simulink library "TOWER_MASTER"  (Simulink 8.8)
settings: Solver=ode45  StartTime=0.0  StopTime=10.0  RelTol=1e-3  EnableMultiTasking=on
undefined symbols (not defined in the file): AC, AC2THRESHOLD, BF_WD_MASTER, GAS_WD_MASTER, GASAC, SIXOSEM_F_WD_AC_MASTER
libraries: cdsEpicsOut x163, cdsFilt x111, cdsTP x68, cdsFiltCtrl x56, cdsEpicsIn x47, cdsMuxMatrix x14, cdsRms x14, TOWER_MASTER x11, STATE_BIO_MASTER x8, cdsEpicsBinIn x6, cdsFunctionCall x4, VIS_LIB x2
(part 2 of 19)

== system TOWER_MASTER/common_blocks/BIOENCODE ==
  note: 1st - 16th bit
  note: 17th bit
  BIO_CTRL_In : Inport
  DIO_OUT : cdsEpicsOut/Subsystem  Tag=cdsEpicsOutput  Description=|
      | Purpose:                                          
      | Output a FE signal to an EPICS channel.           
      |                                                   
      | Operation:                                        
      | Takes input value and passes it to EPICS record.  
      |                                                   
      | Usage:                                            
      | Name the part with the desired EPICS rrecord name.
      settings: AttributesFormatString=%<Tag>
  Gain1 : Gain  Gain=65536
  Ground1 : Ground
  Sum : Sum
  WD_RESET : cdsEpicsBinIn/Subsystem  Tag=cdsEpicsBinIn  Description=|
      | Purpose:                                                                            
      | Create an EPICS binary (0 or 1) input channel to the FE realtime controls.          
      |                                                                                     
      | Operation:                                                                          
      | Outputs value from an EPICS ai record. Value is binary input (bi Epics record type).
      |                                                                                     
      | Usage:                                                                              
      | Name the part with the desired EPICS channel name.
      settings: AttributesFormatString=%<Tag>
  BIO_CTRL_Out : Outport
  wires:
  DIO_OUT/1 -> BIO_CTRL_Out/1
  Sum/1 -> DIO_OUT/1
  BIO_CTRL_In/1 -> Sum/1
  WD_RESET/1 -> Gain1/1
  Ground1/1 -> WD_RESET/1
  Gain1/1 -> Sum/2

== system TOWER_MASTER/common_blocks/GASMASTER ==
  note: #DAQ Channels
      | LVDTINF_GAS_IN1 2048
      | DAMP_GAS_IN1 2048
      | DAMP_GAS_OUT 256
  LVDT_GAS_In : Inport
  MODAL_In : Inport  Port=2
  PEM_SEIS_Z_In : Inport  Port=3
  COILOUT_CTRL : Inport  Port=4
  COILOUTF_MASK : Inport  Port=5
  MASTERSW_In : Inport  Port=6
  WDRESET_In : Inport  Port=7
  BLOCKFLAG : Inport  Port=8
  Modal_IN : Inport  Port=9
  ADD : Subsystem
  COILOUTF : Subsystem
  DAMP : Subsystem
  Demux9 : Demux
  LVDTINF : Subsystem
  MASTER : Subsystem
  Mux9 : Mux  Inputs=2
  SEISFF : Subsystem
  SENSCORR : Subsystem
  SET : Subsystem
  SUMOUT : Subsystem
  Sum1 : Sum  Inputs=++|
  Sum2 : Sum  Inputs=++|
  Sum5 : Sum  Inputs=-+|
  TEST : Subsystem
  Terminator2 : Terminator
  WATCHDOG : cdsFunctionCall/Subsystem  Tag=cdsFunctionCall  Description=inline OSEMWATCHDOG /opt/rtcds/userapps/release/vis/common/src/WATCHDOG.c
      settings: AttributesFormatString=%<Tag>\n%<Description>
  WD : Subsystem
  WDMON : TOWER_MASTER/common_blocks/WDMONMASTER
  GAS_CTR_Out : Outport
  GAS_INF_Out : Outport  Port=2
  WD_STAT_Out : Outport  Port=3
  DAMP_STAT_Out : Outport  Port=4
  wires:
  [FFSTATE] -> Terminator2/1
  SEISFF/1(SEIS_Out) -> ADD/1(SEISFF_In)
  SEISFF/2(SEIS_STATE_Out) -> [FFSTATE]
  PEM_SEIS_Z_In/1 -> SEISFF/1(SEIS_In), SENSCORR/1(SEIS_GAS_In)
  Sum1/1 -> Sum5/2, GAS_INF_Out/1
  SENSCORR/1(SC_GAS_Out) -> Sum1/1
  SET/1(GAS_Out) -> Sum5/1
  Sum5/1 -> DAMP/1(GAS_In)
  MODAL_In/1 -> ADD/2(MODAL_In)
  Demux9/2 -> WDMON/2
  Demux9/3 -> WDMON/3
  WD/1(GAS_AC_FLAG_Out) -> Mux9/2
  COILOUTF/1(Out1) -> MASTER/1(GAS_In)
  LVDTINF/1(Out1) -> Sum1/2
  WATCHDOG/1 -> Demux9/1
  Demux9/4 -> WDMON/4
  Mux9/1 -> WATCHDOG/1
  DAMP/2(DAMP_STATE_Out) -> [DAMPSTATE]
  DAMP/1(GAS_Out) -> ADD/4(DAMP_In)
  MASTERSW_In/1 -> MASTER/2(MASTERSWITCH)
  [WDBLOCKFLAG] -> WD_STAT_Out/1
  [DAMPSTATE] -> DAMP_STAT_Out/1
  TEST/1(GAS_Out) -> ADD/3(TEST_In)
  BLOCKFLAG/1 -> MASTER/3(BLOCKFLAG)
  MASTER/1(GAS_Out) -> GAS_CTR_Out/1
  ADD/1(GAS_MAIN_Out) -> SUMOUT/1(GAS_In)
  Demux9/1 -> WDMON/1, [WDBLOCKFLAG]
  LVDT_GAS_In/1 -> LVDTINF/1(In1), WD/1(GAS_In)
  COILOUT_CTRL/1 -> COILOUTF/2(In2)
  COILOUTF_MASK/1 -> COILOUTF/3(In3)
  WDRESET_In/1 -> Mux9/1
  SUMOUT/1(GAS_Out) -> Sum2/2
  Sum2/1 -> COILOUTF/1(In1)
  Modal_IN/1 -> Sum2/1

== system TOWER_MASTER/common_blocks/OKUTOMIGASMODAL ==
  F0GAS_In : Inport
  F1GAS_In : Inport  Port=2
  F2GAS_In : Inport  Port=3
  F3GAS_In : Inport  Port=4
  BFGAS_In : Inport  Port=5
  ADD : Subsystem
  DAMP : Subsystem
  Demux1 : Demux  Outputs=5
  Demux2 : Demux  Outputs=5
  LVDT2MODAL : cdsMuxMatrix/Subsystem  Tag=cdsMuxMatrix  Description=Any size matrix. Inputs and outputs must be connected using Mux and Demux parts.
      settings: AttributesFormatString=%<Tag>
  MODAL2COIL : cdsMuxMatrix/Subsystem  Tag=cdsMuxMatrix  Description=Any size matrix. Inputs and outputs must be connected using Mux and Demux parts.
      settings: AttributesFormatString=%<Tag>
  MODALOUT : Subsystem
  Mux1 : Mux  Inputs=5
  Mux2 : Mux  Inputs=5
  TEST : Subsystem
  Terminator1 : Terminator
  F0GAS_Out : Outport
  F1GAS_Out : Outport  Port=2
  F2GAS_Out : Outport  Port=3
  F3GAS_Out : Outport  Port=4
  BFGAS_Out : Outport  Port=5
  wires:
  MODALOUT/5(BF_Out) -> BFGAS_Out/1
  MODALOUT/4(F3_Out) -> F3GAS_Out/1
  MODALOUT/3(F2_Out) -> F2GAS_Out/1
  MODALOUT/1(F0_Out) -> F0GAS_Out/1
  MODALOUT/2(F1_Out) -> F1GAS_Out/1
  Demux1/5 -> MODALOUT/5(BF_In)
  Demux1/4 -> MODALOUT/4(F3_In)
  Demux1/3 -> MODALOUT/3(M2_In)
  Demux1/2 -> MODALOUT/2(F1_In)
  Demux1/1 -> MODALOUT/1(F0_In)
  Mux2/1 -> MODAL2COIL/1
  MODAL2COIL/1 -> Demux1/1
  ADD/5(M5_MAIN_Out) -> Mux2/5
  ADD/4(M4_MAIN_Out) -> Mux2/4
  ADD/1(M1_MAIN_Out) -> Mux2/1
  ADD/2(M2_MAIN_Out) -> Mux2/2
  ADD/3(M3_MAIN_Out) -> Mux2/3
  DAMP/1(M1_Out) -> ADD/6(DAMP_M1_In)
  DAMP/5(M5_Out) -> ADD/10(DAMP_M5_In)
  DAMP/2(M2_Out) -> ADD/7(DAMP_M2_In)
  DAMP/4(M4_Out) -> ADD/9(DAMP_M4_In)
  DAMP/3(M3_Out) -> ADD/8(DAMP_M3_In)
  DAMP/6(DAMP_STATE_Out) -> Terminator1/1
  Demux2/2 -> DAMP/2(M2_In)
  Demux2/3 -> DAMP/3(M3_In)
  Demux2/4 -> DAMP/4(M4_In)
  Demux2/1 -> DAMP/1(M1_In)
  Demux2/5 -> DAMP/5(M5_In)
  LVDT2MODAL/1 -> Demux2/1
  TEST/5(M5_Out) -> ADD/5(TEST_M5_In)
  TEST/4(M4_Out) -> ADD/4(TEST_M4_In)
  TEST/3(M3_Out) -> ADD/3(TEST_M3_In)
  TEST/2(M2_Out) -> ADD/2(TEST_M2_In)
  TEST/1(M1_Out) -> ADD/1(TEST_M1_In)
  F1GAS_In/1 -> Mux1/2
  F2GAS_In/1 -> Mux1/3
  BFGAS_In/1 -> Mux1/5
  F0GAS_In/1 -> Mux1/1
  F3GAS_In/1 -> Mux1/4
  Mux1/1 -> LVDT2MODAL/1

== system TOWER_MASTER/common_blocks/OKUTOMIKALMAN ==
  COIL_In1 : Inport
  COIL_In2 : Inport  Port=2
  MEAS_In1 : Inport  Port=3
  MEAS_In2 : Inport  Port=4
  A : cdsMuxMatrix/Subsystem  Tag=cdsMuxMatrix  Description=Any size matrix. Inputs and outputs must be connected using Mux and Demux parts.
      settings: AttributesFormatString=%<Tag>
  ADD_OUTPUT : Subsystem
  ADD_STATE : Subsystem
  B : cdsMuxMatrix/Subsystem  Tag=cdsMuxMatrix  Description=Any size matrix. Inputs and outputs must be connected using Mux and Demux parts.
      settings: AttributesFormatString=%<Tag>
  C : cdsMuxMatrix/Subsystem  Tag=cdsMuxMatrix  Description=Any size matrix. Inputs and outputs must be connected using Mux and Demux parts.
      settings: AttributesFormatString=%<Tag>
  D : cdsMuxMatrix/Subsystem  Tag=cdsMuxMatrix  Description=Any size matrix. Inputs and outputs must be connected using Mux and Demux parts.
      settings: AttributesFormatString=%<Tag>
  Demux{,1..3} (4 alike) : Demux  Outputs=6
  KEST : Subsystem
  Mux : Mux  Inputs=2
  Mux1 : Mux  Inputs=6
  Mux3 : Mux
  UnitDelay{,1..7} (8 alike) : UnitDelay
  Out1 : Outport
  Out2 : Outport  Port=2
  Out3 : Outport  Port=3
  Out4 : Outport  Port=4
  Out5 : Outport  Port=5
  Out6 : Outport  Port=6
  wires:
  KEST/3(X3_Out) -> Out3/1
  KEST/1(X1_Out) -> Out1/1
  KEST/6(X6_Out) -> Out6/1
  KEST/2(X2_Out) -> Out2/1
  KEST/4(X4_Out) -> Out4/1
  KEST/5(X5_Out) -> Out5/1
  ADD_OUTPUT/3(Xest_Out3) -> KEST/3(X3_In)
  ADD_OUTPUT/4(Xest_Out4) -> KEST/4(X4_In)
  ADD_OUTPUT/5(Xest_Out5) -> KEST/5(X5_In)
  ADD_OUTPUT/1(Xest_Out1) -> KEST/1(X1_In)
  ADD_OUTPUT/6(Xest_Out6) -> KEST/6(X6_In)
  ADD_OUTPUT/2(Xest_Out2) -> KEST/2(X2_In)
  MEAS_In2/1 -> Mux3/4
  MEAS_In1/1 -> Mux3/3
  Demux1/6 -> ADD_OUTPUT/12(C_In6)
  Demux1/1 -> ADD_OUTPUT/7(C_In1)
  Demux1/3 -> ADD_OUTPUT/9(C_In3)
  Demux1/2 -> ADD_OUTPUT/8(C_In2)
  Demux1/5 -> ADD_OUTPUT/11(C_In5)
  Demux1/4 -> ADD_OUTPUT/10(C_In4)
  Demux/6 -> ADD_OUTPUT/6(D_In6)
  Demux/3 -> ADD_OUTPUT/3(D_In3)
  Demux/2 -> ADD_OUTPUT/2(D_In2)
  Demux/4 -> ADD_OUTPUT/4(D_In4)
  Demux/5 -> ADD_OUTPUT/5(D_In5)
  Demux/1 -> ADD_OUTPUT/1(D_In1)
  Demux2/5 -> ADD_STATE/11(A_In5)
  Demux2/2 -> ADD_STATE/8(A_In2)
  Demux2/6 -> ADD_STATE/12(A_In6)
  Demux2/3 -> ADD_STATE/9(A_In3)
  Demux2/4 -> ADD_STATE/10(A_In4)
  Demux2/1 -> ADD_STATE/7(A_In1)
  Demux3/2 -> ADD_STATE/2(B_In2)
  Demux3/6 -> ADD_STATE/6(B_In6)
  Demux3/5 -> ADD_STATE/5(B_In5)
  Demux3/4 -> ADD_STATE/4(B_In4)
  Demux3/3 -> ADD_STATE/3(B_In3)
  Demux3/1 -> ADD_STATE/1(B_In1)
  COIL_In1/1 -> UnitDelay1/1, Mux3/1
  COIL_In2/1 -> UnitDelay2/1, Mux3/2
  ADD_STATE/6(dX_Out6) -> UnitDelay7/1
  ADD_STATE/5(dX_Out5) -> UnitDelay6/1
  ADD_STATE/4(dX_Out4) -> UnitDelay5/1
  ADD_STATE/3(dX_Out3) -> UnitDelay4/1
  ADD_STATE/2(dX_Out2) -> UnitDelay3/1
  ADD_STATE/1(dX_Out1) -> UnitDelay/1
  UnitDelay/1 -> Mux1/1
  UnitDelay7/1 -> Mux1/6
  UnitDelay6/1 -> Mux1/5
  UnitDelay3/1 -> Mux1/2
  UnitDelay4/1 -> Mux1/3
  UnitDelay5/1 -> Mux1/4
  UnitDelay1/1 -> Mux/1
  UnitDelay2/1 -> Mux/2
  B/1 -> Demux3/1
  Mux3/1 -> B/1
  A/1 -> Demux2/1
  Mux1/1 -> C/1, A/1
  Mux/1 -> D/1
  C/1 -> Demux1/1
  D/1 -> Demux/1

== system TOWER_MASTER/common_blocks/SHUTDOWNMASTER ==
  WD_Flag : Inport
  BLOCK : cdsEpicsOut/Subsystem  Tag=cdsEpicsOutput  Description=|
      | Purpose:                                          
      | Output a FE signal to an EPICS channel.           
      |                                                   
      | Operation:                                        
      | Takes input value and passes it to EPICS record.  
      |                                                   
      | Usage:                                            
      | Name the part with the desired EPICS rrecord name.
      settings: AttributesFormatString=%<Tag>
  CURRENTTRIG : cdsEpicsOut/Subsystem  Tag=cdsEpicsOutput  Description=|
      | Purpose:                                          
      | Output a FE signal to an EPICS channel.           
      |                                                   
      | Operation:                                        
      | Takes input value and passes it to EPICS record.  
      |                                                   
      | Usage:                                            
      | Name the part with the desired EPICS rrecord name.
      settings: AttributesFormatString=%<Tag>
  Demux : Demux
  FIRSTTRIG : cdsEpicsOut/Subsystem  Tag=cdsEpicsOutput  Description=|
      | Purpose:                                          
      | Output a FE signal to an EPICS channel.           
      |                                                   
      | Operation:                                        
      | Takes input value and passes it to EPICS record.  
      |                                                   
      | Usage:                                            
      | Name the part with the desired EPICS rrecord name.
      settings: AttributesFormatString=%<Tag>
  MODEL_RATE : cdsModelRate/Subsystem  Tag=cdsModelRate
      settings: AttributesFormatString=%<Tag>
  ModWD : cdsFunctionCall/Subsystem  Tag=cdsFunctionCall  Description=inline ModerateWD /opt/rtcds/userapps/release/vis/common/src/ModerateWD.c
      settings: AttributesFormatString=%<Tag>
  Mux : Mux  Inputs=3
  RAMPT : cdsEpicsIn/Subsystem  Tag=cdsEpicsIn  Description=|
      | Purpose:                                                                              
      | Create an EPICS input channel connection to the FE realtime controls.                 
      |                                                                                       
      | Operation:                                                                            
      | Outputs value from an EPICS ai record. Value is floating point with a precision of 3..
      |                                                                                       
      | Usage:                                                                                
      | Name the part with the desired EPICS channel name.
      settings: AttributesFormatString=%<Tag>
  STATE : cdsEpicsOut/Subsystem  Tag=cdsEpicsOutput  Description=|
      | Purpose:                                          
      | Output a FE signal to an EPICS channel.           
      |                                                   
      | Operation:                                        
      | Takes input value and passes it to EPICS record.  
      |                                                   
      | Usage:                                            
      | Name the part with the desired EPICS rrecord name.
      settings: AttributesFormatString=%<Tag>
  Terminator : Terminator
  Terminator1 : Terminator
  Block_Flag : Outport
  State : Outport  Port=2
  wires:
  Mux/1 -> ModWD/1
  ModWD/1 -> Demux/1
  MODEL_RATE/1 -> Mux/3
  BLOCK/1 -> Block_Flag/1
  WD_Flag/1 -> Mux/1
  CURRENTTRIG/1 -> Terminator1/1
  STATE/1 -> State/1
  Demux/3 -> FIRSTTRIG/1
  Demux/4 -> CURRENTTRIG/1
  Demux/2 -> STATE/1
  Demux/1 -> BLOCK/1
  FIRSTTRIG/1 -> Terminator/1
  RAMPT/1 -> Mux/2

== system TOWER_MASTER/common_blocks/WDMONMASTER ==
  BLOCK_Flag : Inport
  STATE_Flag : Inport  Port=2
  FIRST_Flag : Inport  Port=3
  CURRENT_Flag : Inport  Port=4
  BLOCK : cdsEpicsOut/Subsystem  Tag=cdsEpicsOutput  Description="field(PREC,\"3\")"
      settings: AttributesFormatString=%<Tag>
  CURRENTTRIG : cdsEpicsOut/Subsystem  Tag=cdsEpicsOutput  Description="field(PREC,\"3\")"
      settings: AttributesFormatString=%<Tag>
  FIRSTTRIG : cdsEpicsOut/Subsystem  Tag=cdsEpicsOutput  Description="field(PREC,\"3\")"
      settings: AttributesFormatString=%<Tag>
  STATE : cdsEpicsOut/Subsystem  Tag=cdsEpicsOutput  Description="field(PREC,\"3\")"
      settings: AttributesFormatString=%<Tag>
  Terminator{1,3,10..11} (4 alike) : Terminator
  wires:
  STATE_Flag/1 -> STATE/1
  FIRST_Flag/1 -> FIRSTTRIG/1
  CURRENT_Flag/1 -> CURRENTTRIG/1
  CURRENTTRIG/1 -> Terminator11/1
  FIRSTTRIG/1 -> Terminator10/1
  BLOCK_Flag/1 -> BLOCK/1
  BLOCK/1 -> Terminator1/1
  STATE/1 -> Terminator3/1

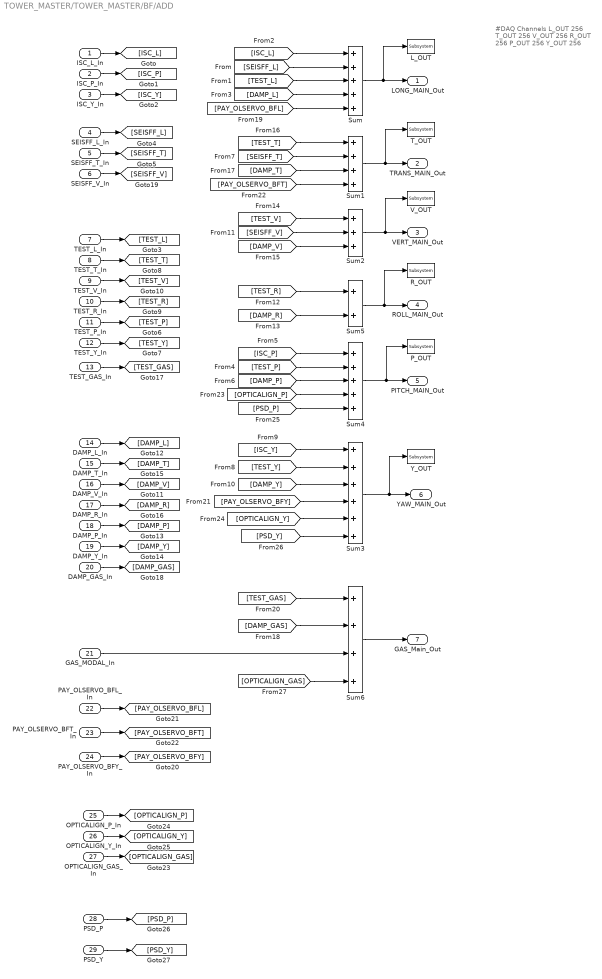
== system TOWER_MASTER/TOWER_MASTER/BF/ADD ==
  note: #DAQ Channels
      |
      | L_OUT 256
      | T_OUT 256
      | V_OUT 256
      | R_OUT 256
      | P_OUT 256
      | Y_OUT 256
  ISC_L_In : Inport
  ISC_P_In : Inport  Port=2
  ISC_Y_In : Inport  Port=3
  SEISFF_L_In : Inport  Port=4
  SEISFF_T_In : Inport  Port=5
  SEISFF_V_In : Inport  Port=6
  TEST_L_In : Inport  Port=7
  TEST_T_In : Inport  Port=8
  TEST_V_In : Inport  Port=9
  TEST_R_In : Inport  Port=10
  TEST_P_In : Inport  Port=11
  TEST_Y_In : Inport  Port=12
  TEST_GAS_In : Inport  Port=13
  DAMP_L_In : Inport  Port=14
  DAMP_T_In : Inport  Port=15
  DAMP_V_In : Inport  Port=16
  DAMP_R_In : Inport  Port=17
  DAMP_P_In : Inport  Port=18
  DAMP_Y_In : Inport  Port=19
  DAMP_GAS_In : Inport  Port=20
  GAS_MODAL_In : Inport  Port=21
  PAY_OLSERVO_BFL_In : Inport  Port=22
  PAY_OLSERVO_BFT_In : Inport  Port=23
  PAY_OLSERVO_BFY_In : Inport  Port=24
  OPTICALIGN_P_In : Inport  Port=25
  OPTICALIGN_Y_In : Inport  Port=26
  OPTICALIGN_GAS_In : Inport  Port=27
  PSD_P : Inport  Port=28
  PSD_Y : Inport  Port=29
  L_OUT : cdsTP/Subsystem  Tag=Test Point
      settings: AttributesFormatString=%<Tag>
  P_OUT : cdsTP/Subsystem  Tag=Test Point
      settings: AttributesFormatString=%<Tag>
  R_OUT : cdsTP/Subsystem  Tag=Test Point
      settings: AttributesFormatString=%<Tag>
  Sum : Sum  Inputs=+++++
  Sum1 : Sum  Inputs=++++
  Sum2 : Sum  Inputs=+++
  Sum3 : Sum  Inputs=++++++
  Sum4 : Sum  Inputs=+++++
  Sum5 : Sum
  Sum6 : Sum  Inputs=++++
  T_OUT : cdsTP/Subsystem  Tag=Test Point
      settings: AttributesFormatString=%<Tag>
  V_OUT : cdsTP/Subsystem  Tag=Test Point
      settings: AttributesFormatString=%<Tag>
  Y_OUT : cdsTP/Subsystem  Tag=Test Point
      settings: AttributesFormatString=%<Tag>
  LONG_MAIN_Out : Outport
  TRANS_MAIN_Out : Outport  Port=2
  VERT_MAIN_Out : Outport  Port=3
  ROLL_MAIN_Out : Outport  Port=4
  PITCH_MAIN_Out : Outport  Port=5
  YAW_MAIN_Out : Outport  Port=6
  GAS_Main_Out : Outport  Port=7
  wires:
  [PAY_OLSERVO_BFT] -> Sum1/4
  [PAY_OLSERVO_BFL] -> Sum/5
  PAY_OLSERVO_BFT_In/1 -> [PAY_OLSERVO_BFT]
  PAY_OLSERVO_BFL_In/1 -> [PAY_OLSERVO_BFL]
  GAS_MODAL_In/1 -> Sum6/3
  [DAMP_GAS] -> Sum6/2
  [TEST_GAS] -> Sum6/1
  [ISC_Y] -> Sum3/1
  [TEST_Y] -> Sum3/2
  [DAMP_Y] -> Sum3/3
  [PAY_OLSERVO_BFY] -> Sum3/4
  [DAMP_P] -> Sum4/3
  [TEST_P] -> Sum4/2
  [SEISFF_V] -> Sum2/2
  [SEISFF_T] -> Sum1/2
  [SEISFF_L] -> Sum/2
  Sum3/1 -> Y_OUT/1, YAW_MAIN_Out/1
  PAY_OLSERVO_BFY_In/1 -> [PAY_OLSERVO_BFY]
  [DAMP_V] -> Sum2/3
  [TEST_V] -> Sum2/1
  [DAMP_T] -> Sum1/3
  [TEST_T] -> Sum1/1
  [DAMP_R] -> Sum5/2
  [TEST_R] -> Sum5/1
  [ISC_P] -> Sum4/1
  ISC_Y_In/1 -> [ISC_Y]
  ISC_P_In/1 -> [ISC_P]
  ISC_L_In/1 -> [ISC_L]
  SEISFF_T_In/1 -> [SEISFF_T]
  SEISFF_L_In/1 -> [SEISFF_L]
  Sum1/1 -> T_OUT/1, TRANS_MAIN_Out/1
  Sum2/1 -> V_OUT/1, VERT_MAIN_Out/1
  Sum5/1 -> R_OUT/1, ROLL_MAIN_Out/1
  [DAMP_L] -> Sum/4
  [TEST_L] -> Sum/3
  [ISC_L] -> Sum/1
  Sum/1 -> L_OUT/1, LONG_MAIN_Out/1
  Sum4/1 -> P_OUT/1, PITCH_MAIN_Out/1
  Sum6/1 -> GAS_Main_Out/1
  SEISFF_V_In/1 -> [SEISFF_V]
  TEST_L_In/1 -> [TEST_L]
  TEST_T_In/1 -> [TEST_T]
  TEST_V_In/1 -> [TEST_V]
  TEST_R_In/1 -> [TEST_R]
  TEST_P_In/1 -> [TEST_P]
  TEST_Y_In/1 -> [TEST_Y]
  TEST_GAS_In/1 -> [TEST_GAS]
  DAMP_L_In/1 -> [DAMP_L]
  DAMP_T_In/1 -> [DAMP_T]
  DAMP_V_In/1 -> [DAMP_V]
  DAMP_R_In/1 -> [DAMP_R]
  DAMP_P_In/1 -> [DAMP_P]
  DAMP_Y_In/1 -> [DAMP_Y]
  DAMP_GAS_In/1 -> [DAMP_GAS]
  OPTICALIGN_Y_In/1 -> [OPTICALIGN_Y]
  OPTICALIGN_P_In/1 -> [OPTICALIGN_P]
  OPTICALIGN_GAS_In/1 -> [OPTICALIGN_GAS]
  PSD_P/1 -> [PSD_P]
  PSD_Y/1 -> [PSD_Y]
  [OPTICALIGN_P] -> Sum4/4
  [PSD_P] -> Sum4/5
  [OPTICALIGN_Y] -> Sum3/5
  [PSD_Y] -> Sum3/6
  [OPTICALIGN_GAS] -> Sum6/4

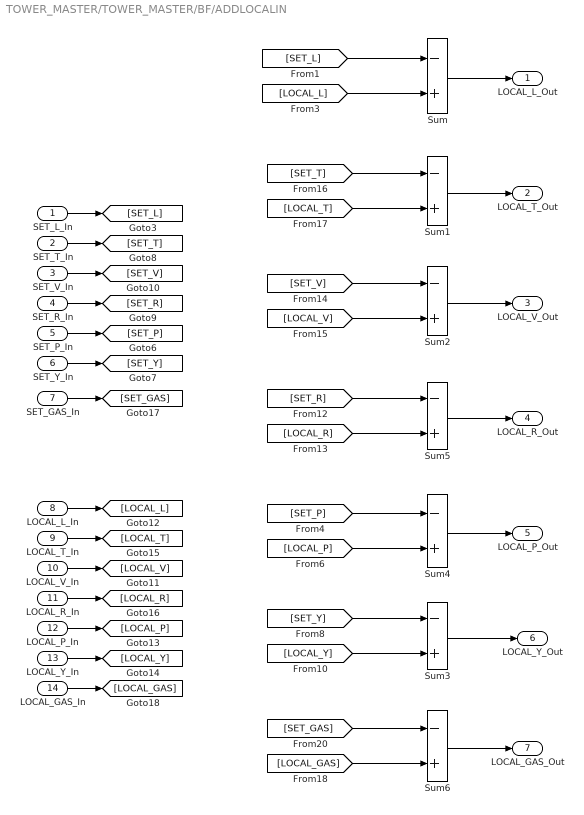
== system TOWER_MASTER/TOWER_MASTER/BF/ADDLOCALIN ==
  SET_L_In : Inport
  SET_T_In : Inport  Port=2
  SET_V_In : Inport  Port=3
  SET_R_In : Inport  Port=4
  SET_P_In : Inport  Port=5
  SET_Y_In : Inport  Port=6
  SET_GAS_In : Inport  Port=7
  LOCAL_L_In : Inport  Port=8
  LOCAL_T_In : Inport  Port=9
  LOCAL_V_In : Inport  Port=10
  LOCAL_R_In : Inport  Port=11
  LOCAL_P_In : Inport  Port=12
  LOCAL_Y_In : Inport  Port=13
  LOCAL_GAS_In : Inport  Port=14
  Sum{,1..6} (7 alike) : Sum  Inputs=-+
  LOCAL_L_Out : Outport
  LOCAL_T_Out : Outport  Port=2
  LOCAL_V_Out : Outport  Port=3
  LOCAL_R_Out : Outport  Port=4
  LOCAL_P_Out : Outport  Port=5
  LOCAL_Y_Out : Outport  Port=6
  LOCAL_GAS_Out : Outport  Port=7
  wires:
  [LOCAL_GAS] -> Sum6/2
  [SET_GAS] -> Sum6/1
  [SET_Y] -> Sum3/1
  [LOCAL_Y] -> Sum3/2
  [SET_P] -> Sum4/1
  [LOCAL_P] -> Sum4/2
  [SET_R] -> Sum5/1
  [LOCAL_R] -> Sum5/2
  [SET_V] -> Sum2/1
  [LOCAL_V] -> Sum2/2
  [SET_T] -> Sum1/1
  [LOCAL_T] -> Sum1/2
  [LOCAL_L] -> Sum/2
  [SET_L] -> Sum/1
  Sum3/1 -> LOCAL_Y_Out/1
  Sum1/1 -> LOCAL_T_Out/1
  Sum2/1 -> LOCAL_V_Out/1
  Sum5/1 -> LOCAL_R_Out/1
  Sum/1 -> LOCAL_L_Out/1
  Sum4/1 -> LOCAL_P_Out/1
  Sum6/1 -> LOCAL_GAS_Out/1
  SET_L_In/1 -> [SET_L]
  SET_T_In/1 -> [SET_T]
  SET_V_In/1 -> [SET_V]
  SET_R_In/1 -> [SET_R]
  SET_P_In/1 -> [SET_P]
  SET_Y_In/1 -> [SET_Y]
  SET_GAS_In/1 -> [SET_GAS]
  LOCAL_L_In/1 -> [LOCAL_L]
  LOCAL_T_In/1 -> [LOCAL_T]
  LOCAL_V_In/1 -> [LOCAL_V]
  LOCAL_R_In/1 -> [LOCAL_R]
  LOCAL_P_In/1 -> [LOCAL_P]
  LOCAL_Y_In/1 -> [LOCAL_Y]
  LOCAL_GAS_In/1 -> [LOCAL_GAS]
